simulink library "hilite_simulink_libs"  (R2024a)
settings: Solver=VariableStepAuto  StartTime=0.0  StopTime=10.0  RelTol=1e-3
libraries: $bdroot x3, simulink x1
settings Model: Creator=ykwang  LastModifiedBy=ykwang

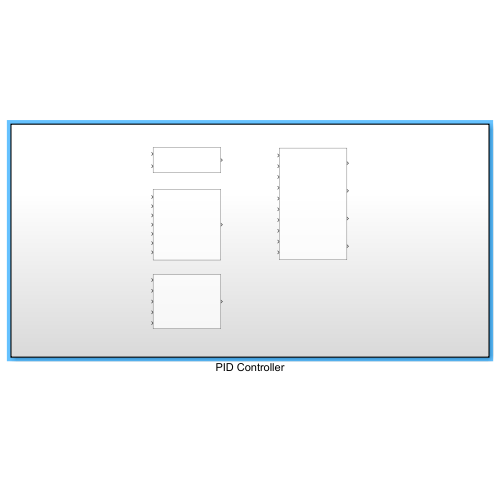
[thumbnail: Simulink's stored preview of the top-level diagram]
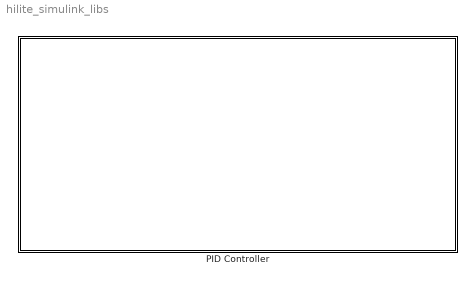
== system hilite_simulink_libs ==
  PID Controller : Subsystem

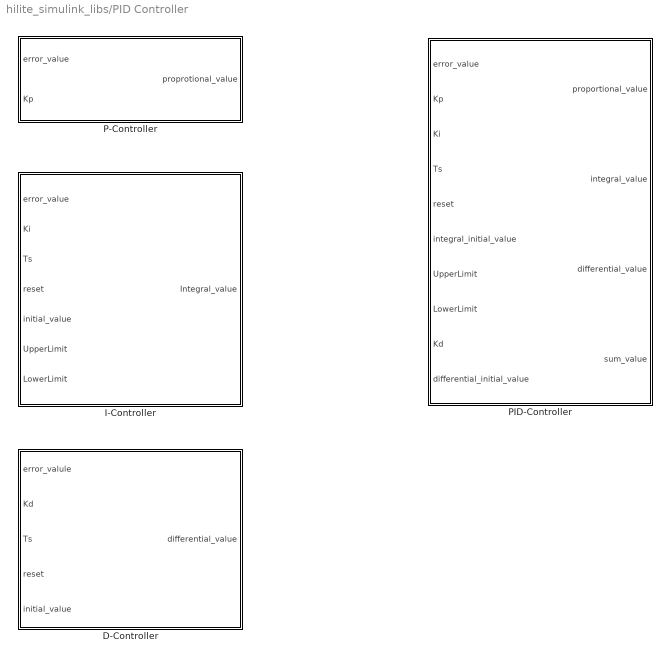
== system hilite_simulink_libs/PID Controller ==
  D-Controller : Subsystem
  I-Controller : Subsystem
  P-Controller : Subsystem
  PID-Controller : Subsystem

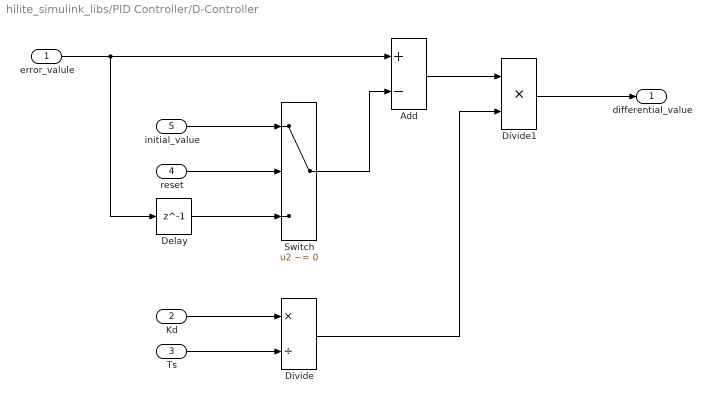
== system hilite_simulink_libs/PID Controller/D-Controller ==
  error_valule : Inport
  Kd : Inport  Port=2
  Ts : Inport  Port=3
  reset : Inport  Port=4
  initial_value : Inport  Port=5
  Add : Sum  Inputs=+-
  Delay : Delay  DelayLength=1
  Divide : Product  Inputs=*/
  Divide1 : Product  Inputs=**
  Switch : Switch  Criteria=u2 ~= 0  SaturateOnIntegerOverflow=off  InputSameDT=off
  differential_value : Outport
  wires:
  error_valule/1 -> Add/1, Delay/1
  Kd/1 -> Divide/1
  Ts/1 -> Divide/2
  Divide/1 -> Divide1/2
  Add/1 -> Divide1/1
  Divide1/1 -> differential_value/1
  reset/1 -> Switch/2
  Delay/1 -> Switch/3
  initial_value/1 -> Switch/1
  Switch/1 -> Add/2

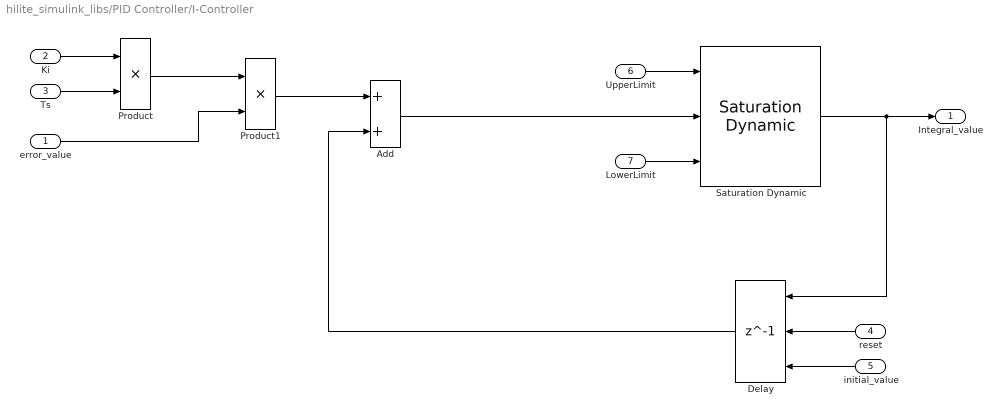
== system hilite_simulink_libs/PID Controller/I-Controller ==
  error_value : Inport
  Ki : Inport  Port=2
  Ts : Inport  Port=3
  reset : Inport  Port=4
  initial_value : Inport  Port=5
  UpperLimit : Inport  Port=6
  LowerLimit : Inport  Port=7
  Add : Sum
  Delay : Delay  DelayLength=1  InitialConditionSource=Input port  InitialCondition=0  ExternalReset=Rising
      settings: InputPortMap=u0,r5,p4
  Product : Product
  Product1 : Product
  Saturation Dynamic : simulink/Discontinuities/Saturation Dynamic  OutMin=[]  OutMax=[]  OutDataTypeStr=Inherit: Same as second input  OutDataType=fixdt(1, 16)  OutScaling=2^-10  DoSatur=off
  Integral_value : Outport
  wires:
  Ki/1 -> Product/1
  Ts/1 -> Product/2
  UpperLimit/1 -> Saturation Dynamic/1
  LowerLimit/1 -> Saturation Dynamic/3
  Saturation Dynamic/1 -> Delay/1, Integral_value/1
  error_value/1 -> Product1/2
  reset/1 -> Delay/2
  Delay/1 -> Add/2
  initial_value/1 -> Delay/3
  Product/1 -> Product1/1
  Product1/1 -> Add/1
  Add/1 -> Saturation Dynamic/2

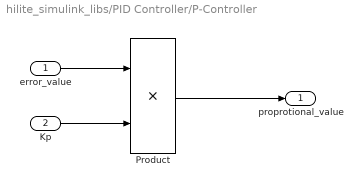
== system hilite_simulink_libs/PID Controller/P-Controller ==
  error_value : Inport
  Kp : Inport  Port=2
  Product : Product
  proprotional_value : Outport
  wires:
  error_value/1 -> Product/1
  Kp/1 -> Product/2
  Product/1 -> proprotional_value/1

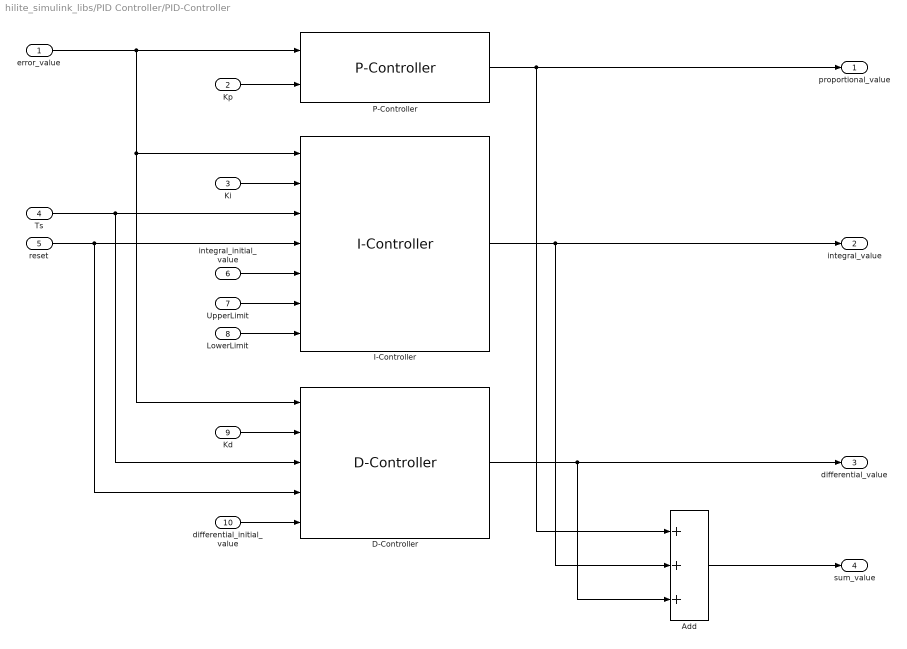
== system hilite_simulink_libs/PID Controller/PID-Controller ==
  error_value : Inport
  Kp : Inport  Port=2
  Ki : Inport  Port=3
  Ts : Inport  Port=4
  reset : Inport  Port=5
  integral_initial_value : Inport  Port=6
  UpperLimit : Inport  Port=7
  LowerLimit : Inport  Port=8
  Kd : Inport  Port=9
  differential_initial_value : Inport  Port=10
  Add : Sum  Inputs=+++
  D-Controller : $bdroot/PID Controller/D-Controller  SystemSampleTime=-1  VariantActivationTime=update diagram  AllowFlexibleInterface=on  Latency=0  AutoFrameSizeCalculation=off
  I-Controller : $bdroot/PID Controller/I-Controller  SystemSampleTime=-1  VariantActivationTime=update diagram  AllowFlexibleInterface=on  Latency=0  AutoFrameSizeCalculation=off
  P-Controller : $bdroot/PID Controller/P-Controller  SystemSampleTime=-1  VariantActivationTime=update diagram  AllowFlexibleInterface=on  Latency=0  AutoFrameSizeCalculation=off
  proportional_value : Outport
  integral_value : Outport  Port=2
  differential_value : Outport  Port=3
  sum_value : Outport  Port=4
  wires:
  error_value/1 -> D-Controller/1, I-Controller/1, P-Controller/1
  Kp/1 -> P-Controller/2
  Ts/1 -> D-Controller/3, I-Controller/3
  Ki/1 -> I-Controller/2
  reset/1 -> D-Controller/4, I-Controller/4
  integral_initial_value/1 -> I-Controller/5
  UpperLimit/1 -> I-Controller/6
  LowerLimit/1 -> I-Controller/7
  P-Controller/1 -> proportional_value/1, Add/1
  I-Controller/1 -> integral_value/1, Add/2
  D-Controller/1 -> Add/3, differential_value/1
  Kd/1 -> D-Controller/2
  differential_initial_value/1 -> D-Controller/5
  Add/1 -> sum_value/1
